simulink model "prob6_week1"  (R2020b)
settings: Solver=VariableStepAuto  StartTime=0.0  StopTime=10.0  RelTol=1e-3
settings Model: Creator=Pulkit Khandelwal  LastModifiedBy=Pulkit Khandelwal

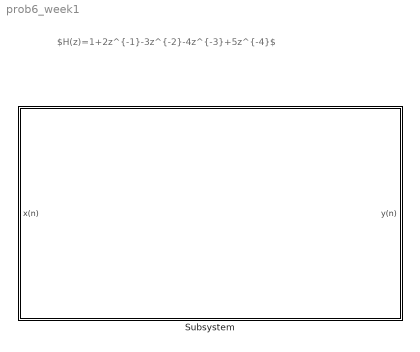
== system prob6_week1 ==
  note: $H(z)=1+2z^{-1}-3z^{-2}-4z^{-3}+5z^{-4}$
  Subsystem : Subsystem  TreatAsAtomicUnit=on

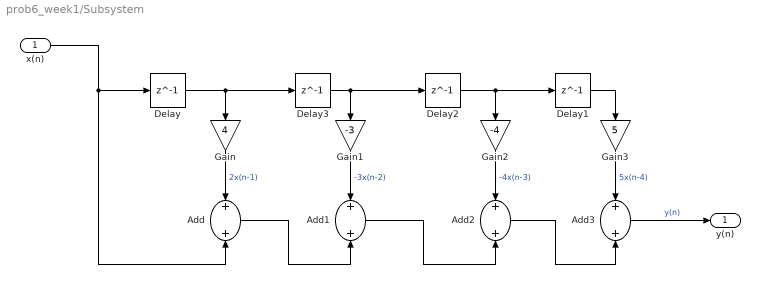
== system prob6_week1/Subsystem ==
  x(n) : Inport
  Add{,1..3} (4 alike) : Sum
  Delay{,1..3} (4 alike) : Delay  DelayLength=1
  Gain : Gain  Gain=4
  Gain1 : Gain  Gain=-3
  Gain2 : Gain  Gain=-4
  Gain3 : Gain  Gain=5
  y(n) : Outport
  wires:
  Delay1/1 -> Gain3/1
  x(n)/1 -> Delay/1, Add/2
  Gain/1 -> Add/1  "2x(n-1)"
  Delay2/1 -> Gain2/1, Delay1/1
  Gain3/1 -> Add3/1  "5x(n-4)"
  Add2/1 -> Add3/2
  Add1/1 -> Add2/2
  Gain2/1 -> Add2/1  "-4x(n-3)"
  Delay/1 -> Delay3/1, Gain/1
  Gain1/1 -> Add1/1  "-3x(n-2)"
  Delay3/1 -> Gain1/1, Delay2/1
  Add/1 -> Add1/2
  Add3/1 -> y(n)/1  "y(n)"
